simulink model "TWC"  (R2022b)
settings: Solver=FixedStepAuto  StartTime=0.0  StopTime=50000000  FixedStep=1  RelTol=1e-3
undefined symbols (not defined in the file): DiscIntNeverNeededParam
libraries: simulink x16
settings Model: Creator=sadamu  LastModifiedBy=程一帆
settings OptimizationCC: DefaultParameterBehavior=Inlined  DefaultUnderspecifiedDataType=single  BufferReuse=off  GlobalBufferReuse=off  ExpressionFolding=off  EnableMemcpy=off  PassReuseOutputArgsAs=Individual arguments  NoFixptDivByZeroProtection=on  EfficientFloat2IntCast=on  OptimizeDataStoreBuffers=off  BusAssignmentInplaceUpdate=off  OptimizationLevel=level0  EfficientTunableParamExpr=on
settings DebuggingCC: ParameterTunabilityLossMsg=error
settings SFSimCC: MATLABDynamicMemAlloc=off
settings RTWCC: Description=Embedded Coder  SystemTargetFile=ert.tlc  GenCodeOnly=on  TemplateMakefile=ert_default_tmf
settings CodeAppCC: ForceParamTrailComments=on  IgnoreCustomStorageClasses=off  OperatorAnnotations=on  SimulinkDataObjDesc=on  SFDataObjDesc=on  InsertBlockDesc=on
settings ERTTargetCC: TargetLangStandard=C99 (ISO)  GenerateSampleERTMain=on  CodeInterfacePackaging=Reusable function  InlinedParameterPlacement=NonHierarchical  ERTCustomFileTemplate=example_file_process.tlc
settings ConfigComp: CovMetricSettings=dcmwe  DVMaxProcessTime=3600  DVTestSuiteOptimization=Auto  DVDetectOutOfBounds=on  DVModelReferenceHarness=on

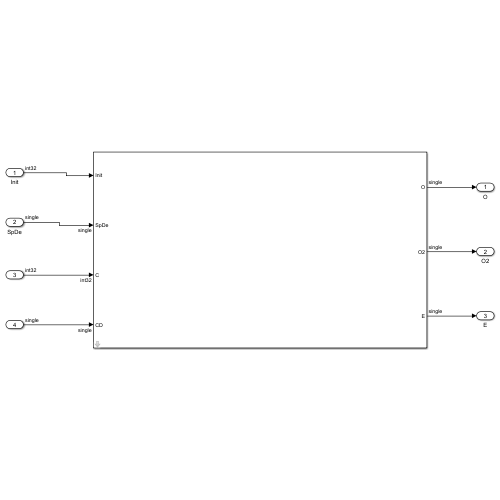
[thumbnail: Simulink's stored preview of the top-level diagram]
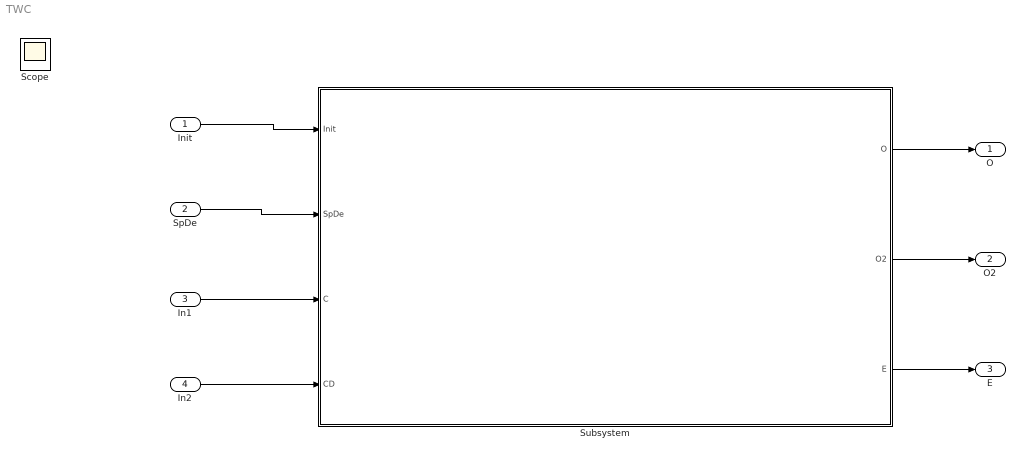
== system TWC ==
  Init : Inport  OutDataTypeStr=int32
  SpDe : Inport  Port=2  OutDataTypeStr=single
  In1 : Inport  Port=3  OutDataTypeStr=int32
  In2 : Inport  Port=4  OutDataTypeStr=single
  Subsystem : Subsystem  mask{Len=32}
      mask DialogControl ParameterGroupVar Prompt: 参数
  O : Outport
  O2 : Outport  Port=2
  E : Outport  Port=3
  Scope : Scope
  wires:
  Init/1 -> Subsystem/1(Init)
  SpDe/1 -> Subsystem/2(SpDe)
  In1/1 -> Subsystem/3(C)
  In2/1 -> Subsystem/4(CD)
  Subsystem/1(O) -> O/1
  Subsystem/2(O2) -> O2/1
  Subsystem/3(E) -> E/1

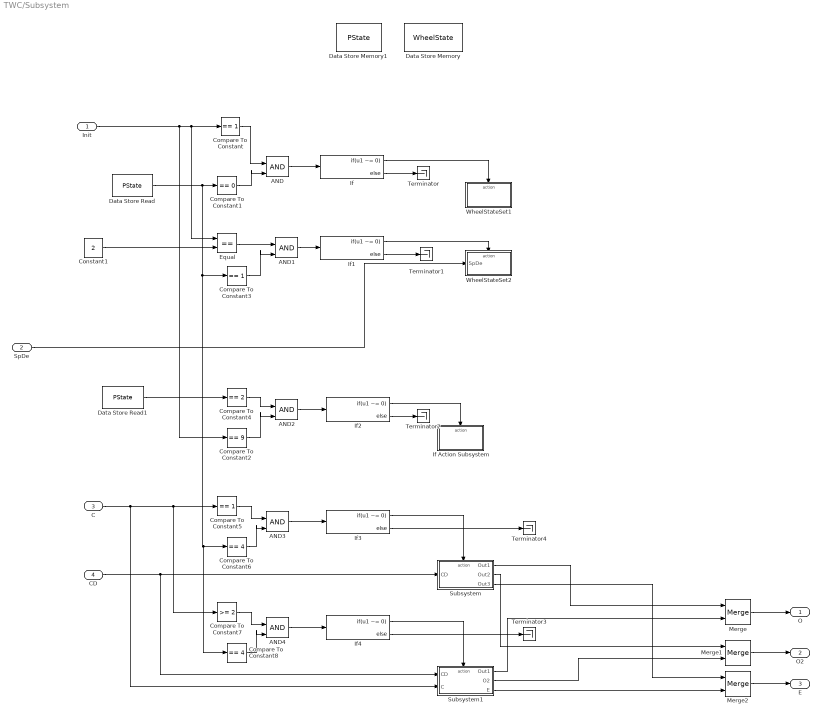
== system TWC/Subsystem ==
  Init : Inport
  SpDe : Inport  Port=2  OutDataTypeStr=single
  C : Inport  Port=3  OutDataTypeStr=int32
  CD : Inport  Port=4  OutDataTypeStr=single
  AND{,1..4} (5 alike) : Logic  IconShape=distinctive  AllPortsSameDT=off  OutDataTypeStr=boolean
  Compare To Constant : simulink/Logic and Bit Operations/Compare To Constant  relop===  const=1  OutDataTypeStr=boolean
  Compare To Constant1 : simulink/Logic and Bit Operations/Compare To Constant  relop===  const=0  OutDataTypeStr=boolean
  Compare To Constant2 : simulink/Logic and Bit Operations/Compare To Constant  relop===  const=9  OutDataTypeStr=boolean
  Compare To Constant3 : simulink/Logic and Bit Operations/Compare To Constant  relop===  const=1  OutDataTypeStr=boolean
  Compare To Constant4 : simulink/Logic and Bit Operations/Compare To Constant  relop===  const=2  OutDataTypeStr=boolean
  Compare To Constant5 : simulink/Logic and Bit Operations/Compare To Constant  relop===  const=1  OutDataTypeStr=boolean
  Compare To Constant6 : simulink/Logic and Bit Operations/Compare To Constant  relop===  const=4  OutDataTypeStr=boolean
  Compare To Constant7 : simulink/Logic and Bit Operations/Compare To Constant  relop=>=  const=2  OutDataTypeStr=boolean
  Compare To Constant8 : simulink/Logic and Bit Operations/Compare To Constant  relop===  const=4  OutDataTypeStr=boolean
  Constant1 : Constant  Value=2  OutDataTypeStr=int32
  Data Store Memory : DataStoreMemory  DataStoreName=WheelState  WriteAfterWriteMsg=warning  ShowAdditionalParam=off  OutDataTypeStr=single  Dimensions=Len
  Data Store Memory1 : DataStoreMemory  DataStoreName=PState  WriteAfterWriteMsg=warning  ShowAdditionalParam=off  OutDataTypeStr=int32
  Data Store Read : DataStoreRead  DataStoreName=PState  IndexOptions=Index vector (dialog)  Indices=1  OutputSizes=1
  Data Store Read1 : DataStoreRead  DataStoreName=PState  IndexOptions=Index vector (dialog)  Indices=1  OutputSizes=1
  Equal : RelationalOperator  Operator===  OutDataTypeStr=boolean  RndMeth=Simplest  InputSameDT=off
  If{,1..4} (5 alike) : If  IfExpression=u1 ~= 0
  If Action Subsystem : Subsystem  TreatAsAtomicUnit=on
  Merge : Merge
  Merge1 : Merge
  Merge2 : Merge
  Subsystem : Subsystem
  Subsystem1 : Subsystem
  Terminator{,1..4} (5 alike) : Terminator
  WheelStateSet1 : Subsystem  TreatAsAtomicUnit=on
  WheelStateSet2 : Subsystem  TreatAsAtomicUnit=on
  O : Outport
  O2 : Outport  Port=2
  E : Outport  Port=3
  wires:
  Compare To Constant/1 -> AND/1
  If/1 -> WheelStateSet1/Action
  Compare To Constant1/1 -> AND/2
  AND/1 -> If/1
  Data Store Read/1 -> Compare To Constant8/1, Compare To Constant6/1, Compare To Constant3/1, Compare To Constant1/1
  If/2 -> Terminator/1
  If1/2 -> Terminator1/1
  Equal/1 -> AND1/1
  AND1/1 -> If1/1
  Compare To Constant3/1 -> AND1/2
  If1/1 -> WheelStateSet2/Action
  SpDe/1 -> WheelStateSet2/1(SpDe)
  AND2/1 -> If2/1
  Compare To Constant2/1 -> AND2/2
  Init/1 -> Compare To Constant2/1, Equal/1, Compare To Constant/1
  Compare To Constant4/1 -> AND2/1
  Data Store Read1/1 -> Compare To Constant4/1
  If2/1 -> If Action Subsystem/Action
  If2/2 -> Terminator2/1
  Constant1/1 -> Equal/2
  C/1 -> Subsystem1/2(C), Compare To Constant7/1, Compare To Constant5/1
  Compare To Constant5/1 -> AND3/1
  Compare To Constant6/1 -> AND3/2
  Subsystem/1(Out1) -> Merge/1
  If3/1 -> Subsystem/Action
  AND3/1 -> If3/1
  Compare To Constant8/1 -> AND4/2
  If4/2 -> Terminator3/1
  CD/1 -> Subsystem1/1(CD), Subsystem/1(CD)
  AND4/1 -> If4/1
  Subsystem1/1(Out1) -> Merge/2
  Compare To Constant7/1 -> AND4/1
  If4/1 -> Subsystem1/Action
  Merge/1 -> O/1
  Subsystem1/2(O2) -> Merge1/2
  Subsystem1/3(E) -> Merge2/2
  Subsystem/2(Out2) -> Merge1/1
  Merge1/1 -> O2/1
  Subsystem/3(Out3) -> Merge2/1
  Merge2/1 -> E/1
  If3/2 -> Terminator4/1

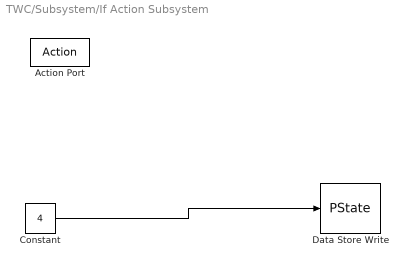
== system TWC/Subsystem/If Action Subsystem ==
  Action Port : ActionPort  ActionPortLabel=if(u1 ~= 0)
  Constant : Constant  Value=4  OutDataTypeStr=int32
  Data Store Write : DataStoreWrite  DataStoreName=PState  IndexOptions=Index vector (dialog)  Indices=1  OutputSizes=1
  wires:
  Constant/1 -> Data Store Write/1

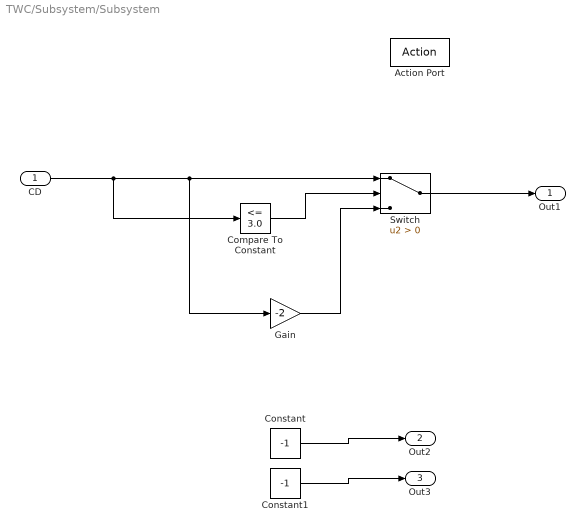
== system TWC/Subsystem/Subsystem ==
  CD : Inport
  Action Port : ActionPort  ActionPortLabel=if(u1 ~= 0)
  Compare To Constant : simulink/Logic and Bit Operations/Compare To Constant  relop=<=  const=3.0  OutDataTypeStr=boolean
  Constant : Constant  Value=-1  OutDataTypeStr=single
  Constant1 : Constant  Value=-1  OutDataTypeStr=single
  Gain : Gain  Gain=-2  OutDataTypeStr=single
  Switch : Switch  Criteria=u2 > Threshold  SaturateOnIntegerOverflow=off  InputSameDT=off
  Out1 : Outport
  Out2 : Outport  Port=2
  Out3 : Outport  Port=3
  wires:
  CD/1 -> Compare To Constant/1, Gain/1, Switch/1
  Gain/1 -> Switch/3
  Compare To Constant/1 -> Switch/2
  Switch/1 -> Out1/1
  Constant/1 -> Out2/1
  Constant1/1 -> Out3/1

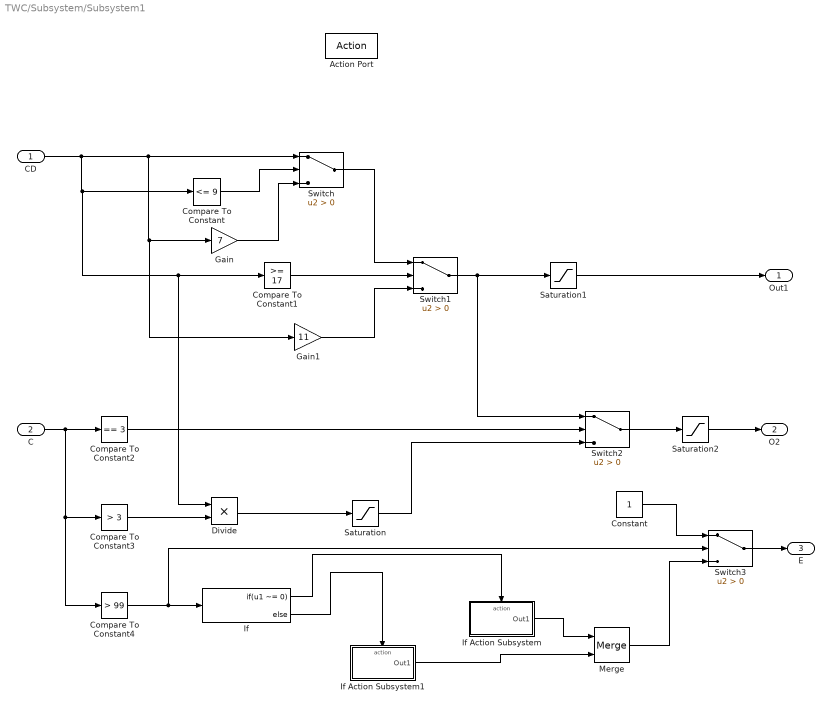
== system TWC/Subsystem/Subsystem1 ==
  CD : Inport
  C : Inport  Port=2
  Action Port : ActionPort  ActionPortLabel=if(u1 ~= 0)
  Compare To Constant : simulink/Logic and Bit Operations/Compare To Constant  relop=<=  const=9  OutDataTypeStr=boolean
  Compare To Constant1 : simulink/Logic and Bit Operations/Compare To Constant  relop=>=  const=17  OutDataTypeStr=boolean
  Compare To Constant2 : simulink/Logic and Bit Operations/Compare To Constant  relop===  const=3  OutDataTypeStr=boolean
  Compare To Constant3 : simulink/Logic and Bit Operations/Compare To Constant  relop=>  const=3  OutDataTypeStr=boolean
  Compare To Constant4 : simulink/Logic and Bit Operations/Compare To Constant  relop=>  const=99  OutDataTypeStr=boolean
  Constant : Constant  OutDataTypeStr=single
  Divide : Product  Inputs=**  OutDataTypeStr=single
  Gain : Gain  Gain=7  OutDataTypeStr=single
  Gain1 : Gain  Gain=11  OutDataTypeStr=single
  If : If  IfExpression=u1 ~= 0
  If Action Subsystem : Subsystem  TreatAsAtomicUnit=on
  If Action Subsystem1 : Subsystem  TreatAsAtomicUnit=on
  Merge : Merge
  Saturation : Saturate  UpperLimit=97  LowerLimit=0
  Saturation1 : Saturate  UpperLimit=97  LowerLimit=0
  Saturation2 : Saturate  UpperLimit=100  LowerLimit=0
  Switch{,1..3} (4 alike) : Switch  Criteria=u2 > Threshold  SaturateOnIntegerOverflow=off  InputSameDT=off
  Out1 : Outport
  O2 : Outport  Port=2
  E : Outport  Port=3
  wires:
  CD/1 -> Divide/1, Compare To Constant1/1, Compare To Constant/1, Gain1/1, Gain/1, Switch/1
  Gain/1 -> Switch/3
  Compare To Constant/1 -> Switch/2
  Switch/1 -> Switch1/1
  Gain1/1 -> Switch1/3
  Compare To Constant1/1 -> Switch1/2
  C/1 -> Compare To Constant4/1, Compare To Constant3/1, Compare To Constant2/1
  Compare To Constant2/1 -> Switch2/2
  Switch2/1 -> Saturation2/1
  Switch1/1 -> Switch2/1, Saturation1/1
  Compare To Constant3/1 -> Divide/2
  Divide/1 -> Saturation/1
  Saturation/1 -> Switch2/3
  Saturation1/1 -> Out1/1
  Saturation2/1 -> O2/1
  Compare To Constant4/1 -> Switch3/2, If/1
  If/1 -> If Action Subsystem/Action
  If/2 -> If Action Subsystem1/Action
  If Action Subsystem/1(Out1) -> Merge/1
  If Action Subsystem1/1(Out1) -> Merge/2
  Merge/1 -> Switch3/3
  Constant/1 -> Switch3/1
  Switch3/1 -> E/1

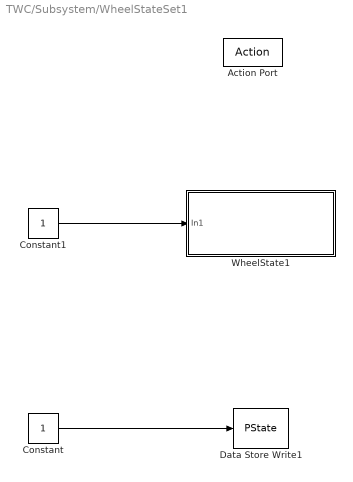
== system TWC/Subsystem/WheelStateSet1 ==
  Action Port : ActionPort  ActionPortLabel=if(u1 ~= 0)
  Constant : Constant  OutDataTypeStr=int32
  Constant1 : Constant  OutDataTypeStr=single
  Data Store Write1 : DataStoreWrite  DataStoreName=PState  IndexOptions=Index vector (dialog)  Indices=1  OutputSizes=1
  WheelState1 : Subsystem  TreatAsAtomicUnit=on
  wires:
  Constant/1 -> Data Store Write1/1
  Constant1/1 -> WheelState1/1(In1)

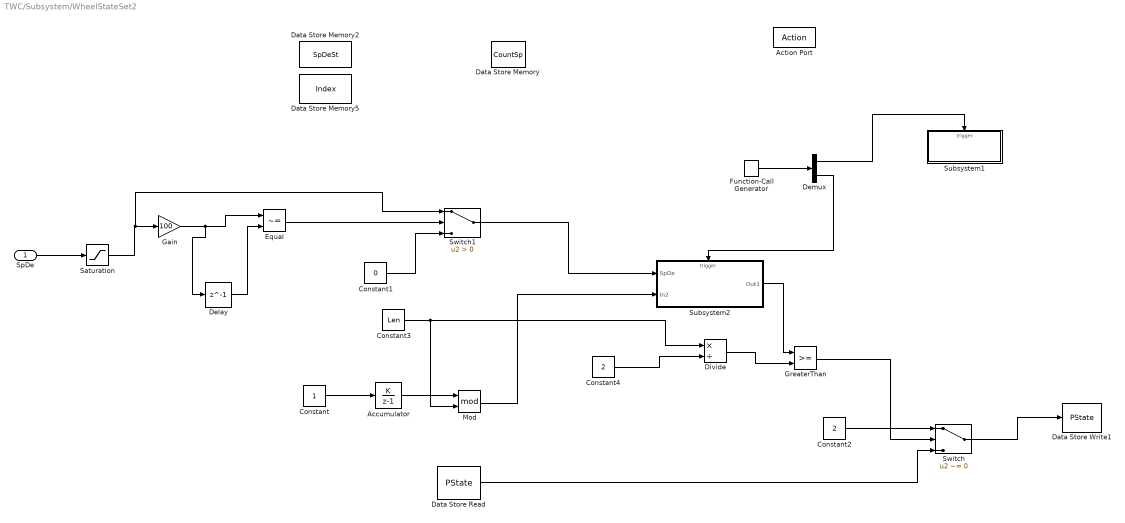
== system TWC/Subsystem/WheelStateSet2 ==
  SpDe : Inport
  Action Port : ActionPort  ActionPortLabel=if(u1 ~= 0)
  Accumulator : DiscreteIntegrator  IntegratorMethod=Accumulation: Forward Euler  SampleTime=-1  ICPrevOutput=DiscIntNeverNeededParam  ICPrevScaledInput=DiscIntNeverNeededParam
  Constant : Constant  OutDataTypeStr=int32
  Constant1 : Constant  Value=0  OutDataTypeStr=single
  Constant2 : Constant  Value=2  OutDataTypeStr=int32
  Constant3 : Constant  Value=Len  OutDataTypeStr=int32
  Constant4 : Constant  Value=2  OutDataTypeStr=int32
  Data Store Memory : DataStoreMemory  DataStoreName=CountSp  WriteAfterWriteMsg=warning  ShowAdditionalParam=off  OutDataTypeStr=int32
  Data Store Memory2 : DataStoreMemory  DataStoreName=SpDeSt  WriteAfterWriteMsg=warning  ShowAdditionalParam=off  OutDataTypeStr=int32  Dimensions=Len
  Data Store Memory5 : DataStoreMemory  DataStoreName=Index  WriteAfterWriteMsg=warning  ShowAdditionalParam=off  OutDataTypeStr=int32
  Data Store Read : DataStoreRead  DataStoreName=PState  IndexOptions=Index vector (dialog)  Indices=1  OutputSizes=1
  Data Store Write1 : DataStoreWrite  DataStoreName=PState  IndexOptions=Index vector (dialog)  Indices=1  OutputSizes=1
  Delay : Delay  DelayLength=1
  Demux : Demux  Outputs=2
  Divide : Product  Inputs=*/
  Equal : RelationalOperator  Operator=~=  OutDataTypeStr=boolean  RndMeth=Simplest  InputSameDT=off
  Function-Call Generator : simulink/Ports & Subsystems/Function-Call Generator  sample_time=1  numberOfIterations=1  DisallowWideOutput=off
  Gain : Gain  Gain=100  OutDataTypeStr=int32
  GreaterThan : RelationalOperator  OutDataTypeStr=boolean  RndMeth=Simplest  InputSameDT=off
  Mod : Math  Operator=mod
  Saturation : Saturate  LowerLimit=0.1
  Subsystem1 : Subsystem
  Subsystem2 : Subsystem
  Switch : Switch  Criteria=u2 ~= 0  SaturateOnIntegerOverflow=off  InputSameDT=off
  Switch1 : Switch  Criteria=u2 > Threshold  SaturateOnIntegerOverflow=off  InputSameDT=off
  wires:
  Constant/1 -> Accumulator/1
  Constant2/1 -> Switch/1
  Mod/1 -> Subsystem2/2(In2)
  SpDe/1 -> Saturation/1
  Saturation/1 -> Switch1/1, Gain/1
  Gain/1 -> Delay/1, Equal/1
  Equal/1 -> Switch1/2
  Constant1/1 -> Switch1/3
  Demux/2 -> Subsystem2/Trigger
  Demux/1 -> Subsystem1/Trigger
  Function-Call Generator/1 -> Demux/1
  Data Store Read/1 -> Switch/3
  Constant3/1 -> Mod/2, Divide/1
  Subsystem2/1(Out1) -> GreaterThan/1
  GreaterThan/1 -> Switch/2
  Switch/1 -> Data Store Write1/1
  Divide/1 -> GreaterThan/2
  Constant4/1 -> Divide/2
  Accumulator/1 -> Mod/1
  Delay/1 -> Equal/2
  Switch1/1 -> Subsystem2/1(SpDe)

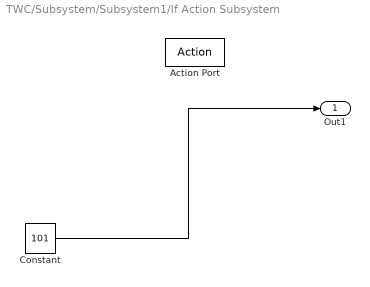
== system TWC/Subsystem/Subsystem1/If Action Subsystem ==
  Action Port : ActionPort  ActionPortLabel=if(u1 ~= 0)
  Constant : Constant  Value=101  OutDataTypeStr=single
  Out1 : Outport
  wires:
  Constant/1 -> Out1/1

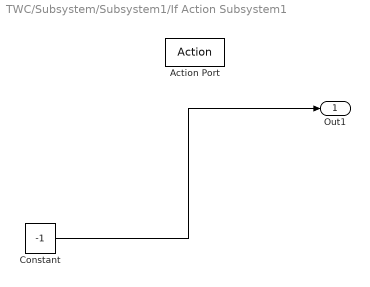
== system TWC/Subsystem/Subsystem1/If Action Subsystem1 ==
  Action Port : ActionPort  ActionPortLabel=else
  Constant : Constant  Value=-1  OutDataTypeStr=single
  Out1 : Outport
  wires:
  Constant/1 -> Out1/1

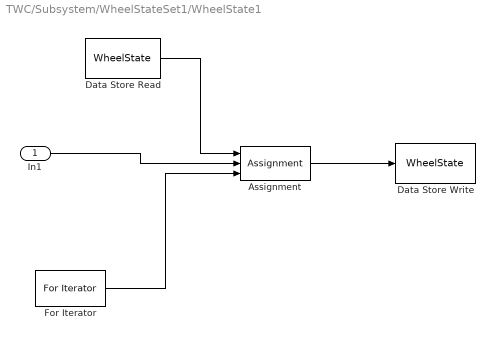
== system TWC/Subsystem/WheelStateSet1/WheelState1 ==
  In1 : Inport
  Assignment : Assignment  IndexMode=Zero-based  DiagnosticForDimensions=Warning  IndexOptions=Index vector (port)  Indices=1  OutputSizes=1
  Data Store Read : DataStoreRead  DataStoreName=WheelState  IndexOptions=Index vector (dialog)  Indices=1  OutputSizes=1
  Data Store Write : DataStoreWrite  DataStoreName=WheelState  IndexOptions=Index vector (dialog)  Indices=1  OutputSizes=1
  For Iterator : ForIterator  IterationLimit=Len  IndexMode=Zero-based
  wires:
  In1/1 -> Assignment/2
  For Iterator/1 -> Assignment/3
  Assignment/1 -> Data Store Write/1
  Data Store Read/1 -> Assignment/1

== system TWC/Subsystem/WheelStateSet2/Subsystem1 ==
  Trigger : TriggerPort  TriggerType=function-call  VariantControl=(inherit)  PortDimensions=1
  Constant : Constant  Value=0  OutDataTypeStr=int32
  Data Store Write : DataStoreWrite  DataStoreName=CountSp  IndexOptions=Index vector (dialog)  Indices=1  OutputSizes=1
  wires:
  Constant/1 -> Data Store Write/1

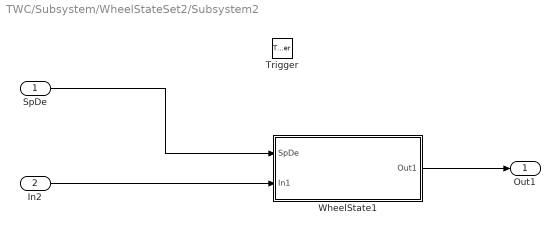
== system TWC/Subsystem/WheelStateSet2/Subsystem2 ==
  SpDe : Inport
  In2 : Inport  Port=2
  Trigger : TriggerPort  TriggerType=function-call  VariantControl=(inherit)  PortDimensions=1
  WheelState1 : Subsystem  TreatAsAtomicUnit=on
  Out1 : Outport
  wires:
  In2/1 -> WheelState1/2(In1)
  SpDe/1 -> WheelState1/1(SpDe)
  WheelState1/1(Out1) -> Out1/1

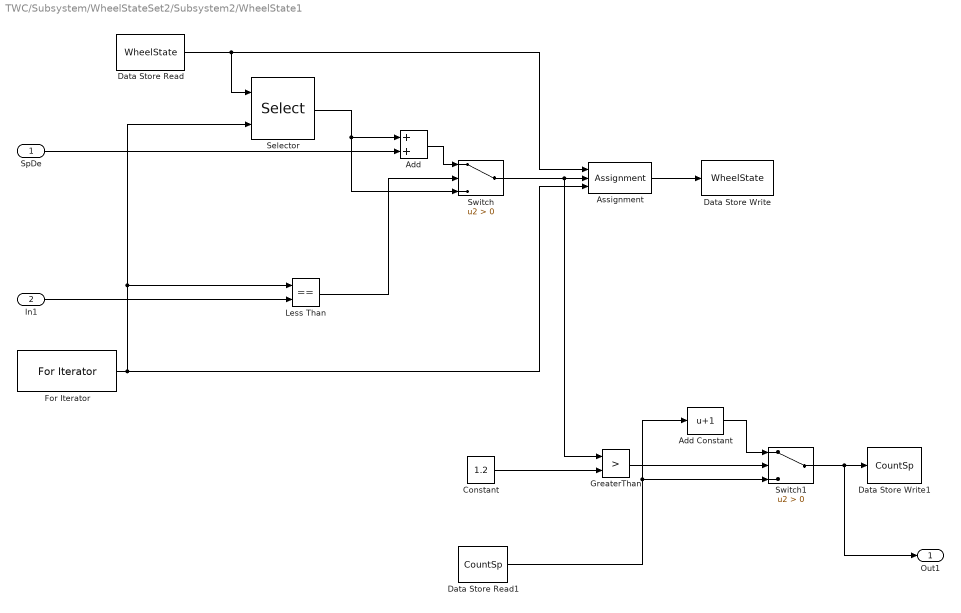
== system TWC/Subsystem/WheelStateSet2/Subsystem2/WheelState1 ==
  SpDe : Inport
  In1 : Inport  Port=2
  Add : Sum
  Add Constant : Bias  Bias=1  SaturateOnIntegerOverflow=off
  Assignment : Assignment  IndexMode=Zero-based  DiagnosticForDimensions=Warning  IndexOptions=Index vector (port)  Indices=1  OutputSizes=1
  Constant : Constant  Value=1.2  OutDataTypeStr=single
  Data Store Read : DataStoreRead  DataStoreName=WheelState  IndexOptions=Index vector (dialog)  Indices=1  OutputSizes=1
  Data Store Read1 : DataStoreRead  DataStoreName=CountSp  IndexOptions=Index vector (dialog)  Indices=1  OutputSizes=1
  Data Store Write : DataStoreWrite  DataStoreName=WheelState  IndexOptions=Index vector (dialog)  Indices=1  OutputSizes=1
  Data Store Write1 : DataStoreWrite  DataStoreName=CountSp  IndexOptions=Index vector (dialog)  Indices=1  OutputSizes=1
  For Iterator : ForIterator  IterationLimit=Len  IndexMode=Zero-based
  GreaterThan : RelationalOperator  Operator=>  OutDataTypeStr=boolean  RndMeth=Simplest  InputSameDT=off
  Less Than : RelationalOperator  Operator===  OutDataTypeStr=boolean  RndMeth=Simplest  InputSameDT=off
  Selector : Selector  IndexMode=Zero-based  InputPortWidth=Len  IndexOptions=Index vector (port)  Indices=[1 3]  OutputSizes=1
  Switch : Switch  Criteria=u2 > Threshold  SaturateOnIntegerOverflow=off  InputSameDT=off
  Switch1 : Switch  Criteria=u2 > Threshold  SaturateOnIntegerOverflow=off  InputSameDT=off
  Out1 : Outport
  wires:
  For Iterator/1 -> Assignment/3, Less Than/1, Selector/2
  Data Store Read/1 -> Selector/1, Assignment/1
  Selector/1 -> Add/1, Switch/3
  Switch/1 -> GreaterThan/1, Assignment/2
  SpDe/1 -> Add/2
  In1/1 -> Less Than/2
  Less Than/1 -> Switch/2
  Assignment/1 -> Data Store Write/1
  Add/1 -> Switch/1
  Constant/1 -> GreaterThan/2
  GreaterThan/1 -> Switch1/2
  Data Store Read1/1 -> Add Constant/1, Switch1/3
  Add Constant/1 -> Switch1/1
  Switch1/1 -> Out1/1, Data Store Write1/1
